simulink model "house_with_pid"  (Simulink 8.4)
settings: Solver=ode45  StartTime=0.0  StopTime=4*3600  RelTol=1e-3
values from neighbouring files (symbols this model uses):
  C_R = 100000    [Simulation.m]
  K = 100    [Simulation.m]
  Q_F_ON = 1000    [Simulation.m]
  Q_H = 1500    [Simulation.m]
  t_a = 0    [Simulation.m]
  t_init = 5    [Simulation.m]
  t_R_set = 20    [Simulation.m]
  tau_F = 2*3600    (= 7200)    [Simulation.m]
  tau_s = 60    [Simulation.m]
libraries: simulink x1, simulink_extras x1
settings Model: Creator=sgt  LastModifiedBy=Admin
settings OptimizationCC: InitFltsAndDblsToZero=on
settings DebuggingCC: SaveWithParameterizedLinksMsg=none  SignalResolutionControl=TryResolveAllWithWarning  MultiTaskDSMMsg=warning  MultiTaskCondExecSysMsg=none
settings RTWCC: IncludeERTFirstTime=on
settings GRTTargetCC: TargetFcnLib=ansi_tfl_tmw.mat

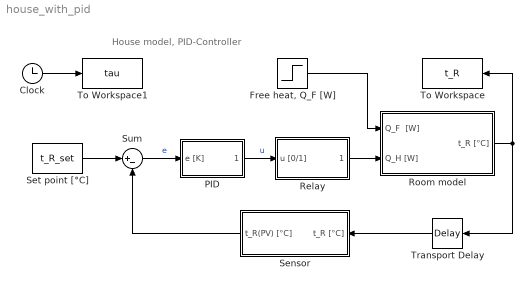
== system house_with_pid ==
  note: House model, PID-Controller
  Clock : Clock
  "Free heat, Q_F [W]" : Step  Time=tau_F  After=Q_F_ON  SampleTime=0
  PID : Subsystem
  Relay : Subsystem
  Room model : Subsystem
  Sensor : Subsystem
  Set point [°C] : Constant  Value=t_R_set
  Sum : Sum  Inputs=|+-
  To Workspace : ToWorkspace  VariableName=t_R  SampleTime=-1
  To Workspace1 : ToWorkspace  VariableName=tau  SampleTime=-1
  Transport Delay : TransportDelay  DelayTime=0
  wires:
  Clock/1 -> To Workspace1/1
  "Free heat, Q_F [W]"/1 -> Room model/1(Q_F  [W])
  Room model/1(t_R [°C]) -> To Workspace/1, Transport Delay/1
  Relay/1(Q_H [W]) -> Room model/2(Q_H [W])
  PID/1(u [0/1]) -> Relay/1(u [0/1])  "u"
  Set point [°C]/1 -> Sum/1
  Sensor/1(t_R(PV) [°C]) -> Sum/2
  Sum/1 -> PID/1(e [K])  "e"
  Transport Delay/1 -> Sensor/1(t_R [°C])

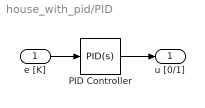
== system house_with_pid/PID ==
  e [K] : Inport
  PID Controller : simulink/Continuous/PID Controller  Controller=PID  TimeDomain=Continuous-time  SampleTime=-1  IntegratorMethod=Forward Euler  FilterMethod=Forward Euler  Form=Parallel  P=1.31115869505421  I=0.00102007570773898  D=45.1755961232093  N=0.0473242120593545  InitialConditionSource=internal  InitialConditionForIntegrator=0  InitialConditionForFilter=0  ExternalReset=none  LimitOutput=off  UpperSaturationLimit=inf  LowerSaturationLimit=-inf  LinearizeAsGain=on  AntiWindupMode=none  Kb=1  TrackingMode=off  Kt=1  PParamMin=[]  PParamMax=[]  IParamMin=[]  IParamMax=[]  DParamMin=[]  DParamMax=[]  NParamMin=[]  NParamMax=[]  KbParamMin=[]  KbParamMax=[]  KtParamMin=[]  KtParamMax=[]  POutMin=[]  POutMax=[]  IOutMin=[]  IOutMax=[]  DOutMin=[]  DOutMax=[]  NOutMin=[]  NOutMax=[]  KbOutMin=[]  KbOutMax=[]  KtOutMin=[]  KtOutMax=[]  IntegratorOutMin=[]  IntegratorOutMax=[]  FilterOutMin=[]  FilterOutMax=[]  SumOutMin=[]  SumOutMax=[]  SumI1OutMin=[]  SumI1OutMax=[]  SumI2OutMin=[]  SumI2OutMax=[]  SumI3OutMin=[]  SumI3OutMax=[]  SumDOutMin=[]  SumDOutMax=[]  SaturationOutMin=[]  SaturationOutMax=[]  IntegratorContinuousStateAttributes=''  IntegratorStateMustResolveToSignalObject=off  IntegratorRTWStateStorageClass=Auto  FilterContinuousStateAttributes=''  FilterStateMustResolveToSignalObject=off  FilterRTWStateStorageClass=Auto  DifferentiatorICPrevScaledInput=0  DifferentiatorOutMin=[]  DifferentiatorOutMax=[]  UseFilter=on
  u [0/1] : Outport
  wires:
  e [K]/1 -> PID Controller/1
  PID Controller/1 -> u [0/1]/1

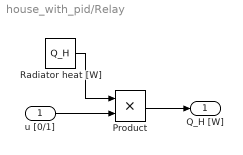
== system house_with_pid/Relay ==
  u [0/1] : Inport
  Product : Product  RndMeth=Zero
  Radiator heat [W] : Constant  Value=Q_H
  Q_H [W] : Outport
  wires:
  Radiator heat [W]/1 -> Product/1
  Product/1 -> Q_H [W]/1
  u [0/1]/1 -> Product/2

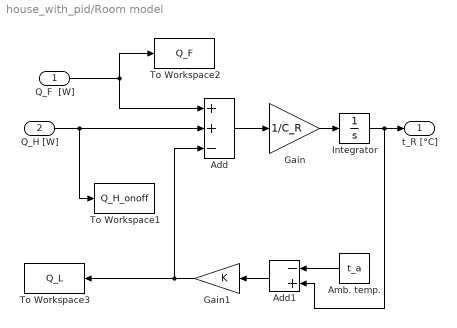
== system house_with_pid/Room model ==
  Q_F  [W] : Inport
  Q_H [W] : Inport  Port=2
  Add : Sum  Inputs=++-
  Add1 : Sum  Inputs=-+
  Amb. temp. : Constant  Value=t_a
  Gain : Gain  Gain=1/C_R
  Gain1 : Gain  Gain=K
  Integrator : Integrator  InitialCondition=t_init
  To Workspace1 : ToWorkspace  VariableName=Q_H_onoff  SampleTime=-1
  To Workspace2 : ToWorkspace  VariableName=Q_F  SampleTime=-1
  To Workspace3 : ToWorkspace  VariableName=Q_L  SampleTime=-1
  t_R [°C] : Outport
  wires:
  Integrator/1 -> Add1/2, t_R [°C]/1
  Gain/1 -> Integrator/1
  Add/1 -> Gain/1
  Q_F  [W]/1 -> To Workspace2/1, Add/1
  Amb. temp./1 -> Add1/1
  Add1/1 -> Gain1/1
  Gain1/1 -> Add/3, To Workspace3/1
  Q_H [W]/1 -> Add/2, To Workspace1/1

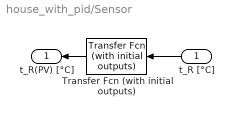
== system house_with_pid/Sensor ==
  t_R [°C] : Inport
  Transfer Fcn (with initial outputs) : simulink_extras/Additional Linear/Transfer Fcn (with initial outputs)  N=[1]  D="[tau_s  1]"  Y0=t_init  U0=0
  t_R(PV) [°C] : Outport
  wires:
  t_R [°C]/1 -> Transfer Fcn (with initial outputs)/1
  Transfer Fcn (with initial outputs)/1 -> t_R(PV) [°C]/1
